simulink model "Main_A"  (R2021a)
settings: Solver=daessc  StartTime=0.0  StopTime=20  RelTol=1e-3
model workspace (MAT data in the model file):
  VEH : object (value not decoded)
values from neighbouring files (symbols this model uses):
  D = 0.15    [Respaldo_ABSfcn.m]
  dT = 0.005    [Init_LightAndPanic70.m]    (also in Init_LowHigh70.m; Init_Panic90.m; Init_Split90.m)
  Mu = [0.93 0.88 0.81 0.86]'    [Init_LightAndPanic70.m]    (also in Init_LowHigh70.m = ones(4,1).*0.9; Init_Panic90.m = ones(4,1).*0.9; Init_Split90.m = ones(4,1).*0.9)
  MuSplit = [0.9 0.4]'    [Init_LightAndPanic70.m]    (also in Init_LowHigh70.m; Init_Panic90.m; Init_Split90.m)
  P_ABSPressureRateMax = 1200    [Init_LightAndPanic70.m]    (also in Init_LowHigh70.m; Init_Panic90.m; Init_Split90.m = 1000)
  P_BrakePressureMax = 120    [Init_LightAndPanic70.m]    (also in Init_LowHigh70.m; Init_Panic90.m; Init_Split90.m)
  P_PedalTravelRateMax = 5    [Init_LightAndPanic70.m]    (also in Init_LowHigh70.m; Init_Panic90.m; Init_Split90.m)
  P_RefLine4SplitMue = 6.14    [Init_LightAndPanic70.m]    (also in Init_LowHigh70.m = 60; Init_Panic90.m; Init_Split90.m)
  P_RefLine_On = false    [Init_LightAndPanic70.m]    (also in Init_LowHigh70.m = true; Init_Panic90.m; Init_Split90.m = true)
  P_RefLineIsX = false    [Init_LightAndPanic70.m]    (also in Init_LowHigh70.m = true; Init_Panic90.m; Init_Split90.m)
  P_SplitMu_On = false    [Init_LightAndPanic70.m]    (also in Init_LowHigh70.m = true; Init_Panic90.m; Init_Split90.m = true)
  P_SplitMuOnlyAtBraking = false    [Init_LightAndPanic70.m]    (also in Init_LowHigh70.m = true; Init_Panic90.m; Init_Split90.m = true)
  P_SteeringMax = 20    [Init_LightAndPanic70.m]    (also in Init_LowHigh70.m; Init_Panic90.m; Init_Split90.m)
  P_TorqueMax = 600    [Init_LightAndPanic70.m]    (also in Init_LowHigh70.m; Init_Panic90.m; Init_Split90.m)
  t_Brake = 9    [Init_LightAndPanic70.m]    (also in Init_LowHigh70.m = 12; Init_Panic90.m = 12; Init_Split90.m = 12)
symbols that are objects in the model workspace (value not decoded): VEH
libraries: sim3dlib x2, simulink_extras x1, vehdynlibsteering x1, sim3dautolib x1, simulink x1, vehdynlibviscommon x1
(part 2 of 2)

== matlab function Main_A/Environment/EnhancedSplitMu/SplitMu Function ==
  data: VehDim input; X input; mu_FL output; Y input; psi input; SplitMu input; SplitLine input; mu_FR output; mu_RL output; mu_RR output; XorY input
function [mu_FL,mu_FR,mu_RL,mu_RR] = fcn(VehDim,X,Y,psi,SplitMu,SplitLine,XorY)

% Right-hand rule ******************************************************* %
%   X                                                                     %
%   |             - X-axis aligns with vehicle's longitudinal axis        %
%   |             - Z-axis points downwards                               %
%   |_ _ _ _ Y                                                            %
% *********************************************************************** %

% Vehicle dimensions
TW2   = VehDim(1)/2;   % Track width divided by 2
CG2FA = VehDim(2);     % Distance from CG to front axle
CG2RA = VehDim(3);     % Distance from CG to rear axle

% Inertial frame coordinates
CG = [X; Y];           % Location of the vehicle in the inertial frame

% Vehicle's body frame coordinates [x; y]
CG2FL = [ CG2FA; -TW2];
CG2FR = [ CG2FA;  TW2];
CG2RL = [-CG2RA; -TW2];
CG2RR = [-CG2RA;  TW2];

% Rotation matrix
R = [cos(psi), -sin(psi);...
     sin(psi),  cos(psi)];

% Coordinate transformation of body frame to inertial frame
O_FL = R * CG2FL + CG;
O_FR = R * CG2FR + CG;
O_RL = R * CG2RL + CG;
O_RR = R * CG2RR + CG;

% Mu selection for each wheel based on the "surface" they are on.
% Each vector follows the definition [FL; FR; RL; RR]
if XorY == true
    temp = 1;
else
    temp = 2;
end
O_split = [O_FL(temp); O_FR(temp); O_RL(temp); O_RR(temp)];
Mu   = zeros(4,1);

for i = 1:4
    if O_split(i) < SplitLine
        Mu(i) = SplitMu(1);
    else
        Mu(i) = SplitMu(2);
    end
end

mu_FL = Mu(1);
mu_FR = Mu(2);
mu_RL = Mu(3);
mu_RR = Mu(4);

end

== matlab function Main_A/BrakeController/ECU ==
  data: Enable input; dT input; pMC input; WSS input; IMU input; pWhl output; MEM input; MEM_out output; Vel output; Desl output; YawRate output; LatAcc output; Yaw output; control output; t output; Velmax output; d output
function [pWhl, MEM_out,Vel,Desl,YawRate,LatAcc,Yaw,control,t,Velmax,d]= fcn(Enable, dT, pMC, WSS, IMU, MEM)

% ****************************** IMPORTANT ****************************** %
% NO work has to be done here. NO need to change this script, unless you
% need a different interface (i.e. inputs/outputs) to design or debug your
% controller.
% This function block only serves as a bridge to ABSfcn.m, so the
% controller's script (ABSfcn.m) can be stored in a file independent from
% the simulink model.
% *********************************************************************** %

% ******************************* INPUTS: ******************************* %
% Enable --> Switch to enable/disable controller (logic bit)              %
% Refer to ABSfcn.m for details regarding the rest of inputs              %
% *********************************************************************** %

% ************************ CASE: PASSIVE BRAKING ************************ %
% Passive braking means no control, whatsoever. Master cylinder pressure  %
% is equally passed to all wheels, same brake pressure across the         %
% multiple brake lines.                                                   %
if not(Enable)
    [pWhl, MEM_out,Vel,Desl,YawRate,LatAcc,Yaw,control,t,Velmax,d] = ABSfcn(dT, pMC, WSS, IMU, MEM);
    
    
    
    pWhl    = [pMC pMC pMC pMC]';
    %MEM_out = zeros(50,1);
    
    return; % Exit function and do not run the rest of lines
end
% ********************* CASE: PASSIVE BRAKING - END ********************* %


% ********************** CASE: ABS CONTROL ENABLED ********************** %
[pWhl, MEM_out,Vel,Desl,YawRate,LatAcc,Yaw,control,t,Velmax,d] = ABSfcn(dT, pMC, WSS, IMU, MEM);
% ******************* CASE: ABS CONTROL ENABLED - END ******************* %

end
